simulink model "Final_updated1_backup_final"  (R2018b)
settings: Solver=ode45  StartTime=0.0  StopTime=10.0  RelTol=1e-3
libraries: powerlib x12, powerlib_meascontrol x1
settings Model: Creator=Vishnu Ajith  LastModifiedBy=Vishnu Ajith

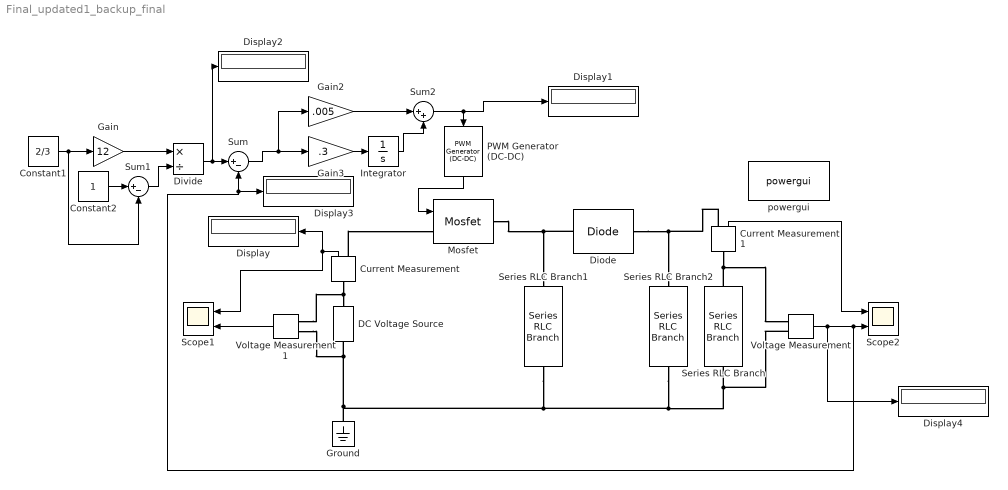
== system Final_updated1_backup_final ==
  Constant1 : Constant  Value=2/3
  Constant2 : Constant
  Current Measurement : powerlib/Measurements/Current Measurement  PhasorSimulation=off  OutputType=Complex  PSBequivalent=0
  Current Measurement1 : powerlib/Measurements/Current Measurement  PhasorSimulation=off  OutputType=Complex  PSBequivalent=0
  DC Voltage Source : powerlib/Electrical Sources/DC Voltage Source  Amplitude=12  Measurements=Voltage
  Diode : powerlib/Power Electronics/Diode  Ron=1e-3  Lon=0  Vf=0.8  IC=0  UseSnubber=0  Rs=inf  Cs=inf  Measurements=off
  Display{,1..4} (5 alike) : Display
  Divide : Product  Inputs=*/
  Gain : Gain  Gain=12
  Gain2 : Gain  Gain=.005
  Gain3 : Gain  Gain=.3
  Ground : powerlib/Elements/Ground  LConnTagsString=a
  Integrator : Integrator  ZeroCross=off
  Mosfet : powerlib/Power Electronics/Mosfet  Ron=0.1  Lon=0  Rd=0.01  Vfd=0  IC=0  Rs=1e6  Cs=inf  Measurements=off
  PWM Generator (DC-DC) : powerlib_meascontrol/Pulse & Signal Generators/PWM Generator (DC-DC)  Fsw=10000  Ts=0
  Scope1 : Scope  NumInputPorts=2
  Scope2 : Scope  NumInputPorts=2
  Series RLC Branch : powerlib/Elements/Series RLC Branch  LConnTagsString=__new0  RConnTagsString=__new0  BranchType=R  Resistance=50  Inductance=1e-3  SetiL0=off  InitialCurrent=0  Capacitance=1e-6  Setx0=off  InitialVoltage=0  Measurements=Branch voltage and current
  Series RLC Branch1 : powerlib/Elements/Series RLC Branch  LConnTagsString=__new0  RConnTagsString=__new0  BranchType=L  Resistance=1  Inductance=2.23e-3  SetiL0=off  InitialCurrent=0  Capacitance=1e-6  Setx0=off  InitialVoltage=0  Measurements=None
  Series RLC Branch2 : powerlib/Elements/Series RLC Branch  LConnTagsString=__new0  RConnTagsString=__new0  BranchType=C  Resistance=1  Inductance=1e-3  SetiL0=off  InitialCurrent=0  Capacitance=100e-5  Setx0=off  InitialVoltage=0  Measurements=None
  Sum : Sum  Inputs=|+-
  Sum1 : Sum  Inputs=|+-
  Sum2 : Sum  Inputs=|++
  Voltage Measurement : powerlib/Measurements/Voltage Measurement  PhasorSimulation=off  OutputType=Complex  PSBequivalent=0
  Voltage Measurement1 : powerlib/Measurements/Voltage Measurement  PhasorSimulation=off  OutputType=Complex  PSBequivalent=0
  powergui : powerlib/powergui  Priority=1  SimulationMode=Discrete  SampleTime=1e-6  frequency=60  Iterations=50  frequencyindice=0  Pbase=100e6  ErrMax=1e-4  UnitsV=kV  UnitsW=MW  buscounter=0  FunctionMessages=off  echomessages=off  EnableUseOfTLC=off  CurrentSourceSwitches=off  DisableSnubberDevices=off  DisableRonSwitches=off  DisableVfSwitches=off  DisplayEquations=off  SolverType=Tustin/Backward Euler (TBE)  Interpol=off  ExternalGateDelay=off  methode=off  Ts=100  x0status=blocks  SPID=on  SwTol=0  HookPort=off  RestoreLinks=warning  ResistiveCurrentMeasurement=off  Frange=[0:2:500]  Ylog=off  Xlog=on  ShowGrid=off  save=off  variable=ZData  structure=0  ZoomFFT=off  StartTime=0.0  cycles=1  DisplayStyle=1  fundamental=60  FreqAxis=off  MaxFrequency=1000  frequencyindicesteady=1  RmsSteady=1  display=off
  wires:
  Current Measurement/1 -> Scope1/1, Display/1
  Current Measurement1/1 -> Scope2/1
  Voltage Measurement/1 -> Display4/1, Display3/1, Sum/2, Scope2/2
  Voltage Measurement1/1 -> Scope1/2
  Constant1/1 -> Sum1/2, Gain/1
  Divide/1 -> Display2/1, Sum/1
  Gain/1 -> Divide/1
  Sum1/1 -> Divide/2
  Constant2/1 -> Sum1/1
  PWM Generator (DC-DC)/1 -> Mosfet/1
  Gain3/1 -> Integrator/1
  Gain2/1 -> Sum2/1
  Integrator/1 -> Sum2/2
  Sum2/1 -> Display1/1, PWM Generator (DC-DC)/1
  Sum/1 -> Gain2/1, Gain3/1
  connections:
  Current Measurement/LConn1 -- DC Voltage Source/RConn1 -- Voltage Measurement1/LConn1
  Mosfet/RConn1 -- Diode/RConn1 -- Series RLC Branch1/LConn1
  Diode/LConn1 -- Current Measurement1/RConn1 -- Series RLC Branch2/LConn1
  Series RLC Branch2/RConn1 -- Series RLC Branch1/RConn1 -- Voltage Measurement1/LConn2 -- DC Voltage Source/LConn1 -- Ground/LConn1 -- Voltage Measurement/LConn1 -- Series RLC Branch/RConn1
  Current Measurement/RConn1 -- Mosfet/LConn1
  Series RLC Branch/LConn1 -- Voltage Measurement/LConn2 -- Current Measurement1/LConn1
